simulink model "hw1_q4_lypunov_adaptive"  (R2021a)
settings: Solver=VariableStepAuto  StartTime=0.0  StopTime=10.0  RelTol=1e-3
settings Model: Creator=chint  LastModifiedBy=chint

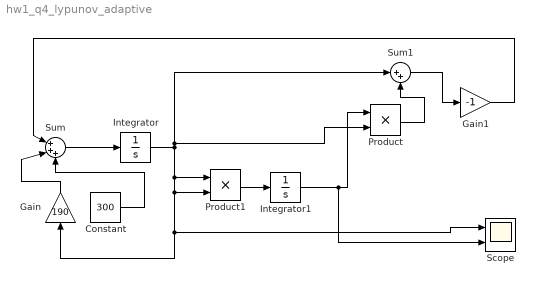
== system hw1_q4_lypunov_adaptive ==
  Constant : Constant  Value=300
  Gain : Gain  Gain=190
  Gain1 : Gain  Gain=-1
  Integrator : Integrator  InitialCondition=100
  Integrator1 : Integrator
  Product : Product
  Product1 : Product
  Scope : Scope  NumInputPorts=2
  Sum : Sum  Inputs=|+++
  Sum1 : Sum  Inputs=|++
  wires:
  Sum/1 -> Integrator/1
  Gain/1 -> Sum/2
  Integrator/1 -> Sum1/1, Product/2, Product1/1, Product1/2, Scope/1, Gain/1
  Product1/1 -> Integrator1/1
  Integrator1/1 -> Scope/2, Product/1
  Gain1/1 -> Sum/1
  Product/1 -> Sum1/2
  Sum1/1 -> Gain1/1
  Constant/1 -> Sum/3
